simulink model "Digflt"  (Simulink 3.00)
settings: Solver=ode45  StartTime=0.0  StopTime=10.0  RelTol=1e-3
libraries: Dequiv x15, simulink3 x1
settings Model: LastModifiedBy=campa

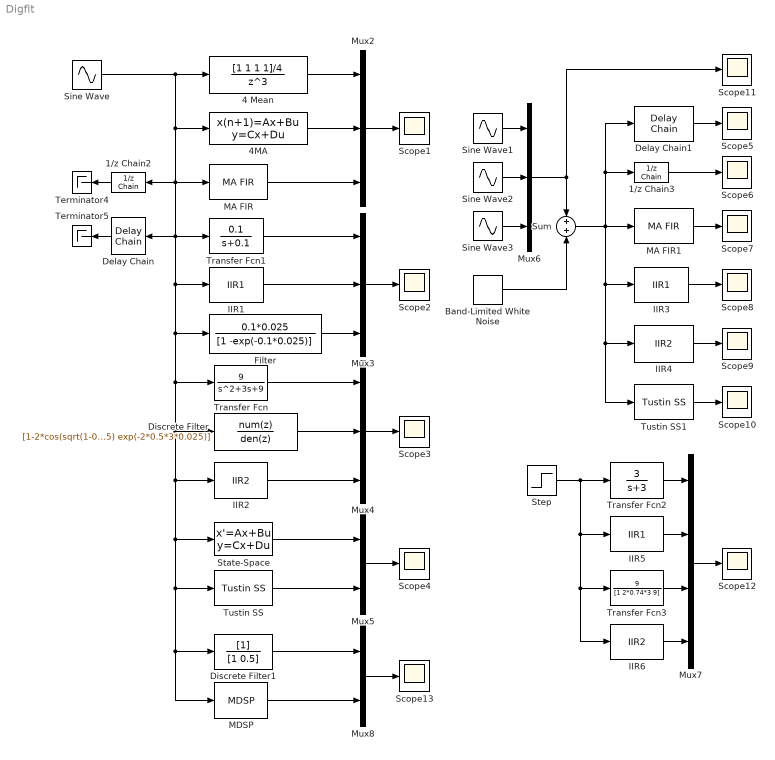
== system Digflt ==
  1/z Chain2 : Dequiv/1//z Chain  Orientation=left  ni=1  rd=4  x0=0  T=0.025
  1/z Chain3 : Dequiv/1//z Chain  ni=3  rd=4  x0=0  T=0.025
  4 Mean : DiscreteTransferFcn  Numerator=[1 1 1 1]/4  Denominator=[1 0 0 0]  SampleTime=0.025
  4MA : DiscreteStateSpace  A=[0 1 0;0 0 1;0 0 0]  B=[0 0 1/4]'  C=[1 1 1]  D=1/4  X0=0  SampleTime=0.025
  Band-Limited White Noise : simulink3/Sources/Band-Limited White Noise  Cov=0.01*ones(3,1)  Ts=0.025  seed=[1 2 3]
  Delay Chain : Dequiv/Delay Chain  Orientation=left  ni=1  rd=3  x0=2e-7/4  T=0.025
  Delay Chain1 : Dequiv/Delay Chain  ni=3  rd=3  x0=2e-7/4  T=0.025
  Discrete Filter : DiscreteFilter  Numerator=[1-2*cos(sqrt(1-0.5^2)*3*0.025)*exp(-0.5*3*0.025)+exp(-2*0.5*3*0.025)]  Denominator=[1 -2*cos(sqrt(1-0.5^2)*3*0.025)*exp(-0.5*3*0.025) exp(-2*0.5*3*0.025)]  SampleTime=0.025
  Discrete Filter1 : DiscreteFilter  Numerator=[1]  Denominator=[1 0.5]  SampleTime=0.025
  Filter : DiscreteFilter  Numerator=0.1*0.025  Denominator=[1 -exp(-0.1*0.025)]  SampleTime=0.025
  IIR1 : Dequiv/IIR1  ni=1  a=0.1  x0=0  T=0.025
  IIR2 : Dequiv/IIR2  ni=1  w=3  x=0.5  x0=0  T=0.025
  IIR3 : Dequiv/IIR1  ni=3  a=3  x0=0  T=0.025
  IIR4 : Dequiv/IIR2  ni=3  w=3  x=0.74  x0=0  T=0.025
  IIR5 : Dequiv/IIR1  ni=1  a=3  x0=0  T=0.025
  IIR6 : Dequiv/IIR2  ni=1  w=3  x=0.74  x0=0  T=0.025
  MA FIR : Dequiv/MA FIR  ni=1  ws=4  x0=2e-7/4  T=0.025
  MA FIR1 : Dequiv/MA FIR  ni=3  ws=4  x0=2e-7/4  T=0.025
  MDSP : Dequiv/MDSP  ni=1  num=[1 0]  den=[1 0.5]  u0=0  T=0.025
  Mux{2..4,6} (4 alike) : Mux  Inputs=3
  Mux5 : Mux  Inputs=2
  Mux7 : Mux  Inputs=4
  Mux8 : Mux  Inputs=2
  Scope{1..13} (13 alike) : Scope
      Scope1 settings: TimeRange=10  YMin=-1  YMax=1  SaveToWorkspace=off  SaveName=ScopeData
      Scope10 settings: TimeRange=10  YMin=-1  YMax=1  SaveToWorkspace=off  SaveName=ScopeData
      Scope11 settings: TimeRange=10  YMin=-1  YMax=1  SaveToWorkspace=off  SaveName=ScopeData
      Scope12 settings: TimeRange=10  YMin=0  YMax=1.5  SaveToWorkspace=off  SaveName=ScopeData
      Scope13 settings: TimeRange=10  YMin=-1  YMax=1  SaveToWorkspace=off  SaveName=ScopeData
      Scope2 settings: TimeRange=10  YMin=-0.05  YMax=0.15  SaveToWorkspace=off  SaveName=ScopeData
      Scope3 settings: TimeRange=10  YMin=-2  YMax=2  SaveToWorkspace=off  SaveName=ScopeData
      Scope4 settings: TimeRange=10  YMin=-1  YMax=1  SaveToWorkspace=off  SaveName=ScopeData
      Scope5 settings: TimeRange=10  YMin=-4  YMax=4  SaveToWorkspace=off  SaveName=ScopeData
      Scope6 settings: TimeRange=10  YMin=-4  YMax=4  SaveToWorkspace=off  SaveName=ScopeData
      Scope7 settings: TimeRange=10  YMin=-2  YMax=2  SaveToWorkspace=off  SaveName=ScopeData
      Scope8 settings: TimeRange=10  YMin=-1  YMax=1  SaveToWorkspace=off  SaveName=ScopeData
      Scope9 settings: TimeRange=10  YMin=-1  YMax=1  SaveToWorkspace=off  SaveName=ScopeData
  Sine Wave : Sin  Amplitude=1  Frequency=2  Phase=0  SampleTime=0
  Sine Wave1 : Sin  Amplitude=1  Frequency=1.5  Phase=0  SampleTime=0
  Sine Wave2 : Sin  Amplitude=1  Frequency=1.5  Phase=pi/4  SampleTime=0
  Sine Wave3 : Sin  Amplitude=1  Frequency=1.5  Phase=pi/2  SampleTime=0
  State-Space : StateSpace  A=[0 1;-3^2 -2*3*0.74]  B=[0;3^2]  C=[1 0]  D=0  X0=0
  Step : Step  Time=1  Before=0  After=1  SampleTime=0
  Sum : Sum  Inputs=++  SaturateOnIntegerOverflow=on
  Terminator4 : Terminator
  Terminator5 : Terminator
  Transfer Fcn : TransferFcn  Numerator=9  Denominator=[1 3 9]
  Transfer Fcn1 : TransferFcn  Numerator=0.1  Denominator=[1 0.1]
  Transfer Fcn2 : TransferFcn  Numerator=3  Denominator=[1 3]
  Transfer Fcn3 : TransferFcn  Numerator=9  Denominator=[1 2*0.74*3 9]
  Tustin SS : Dequiv/Tustin SS  n=1  a=[0 1;-3^2 -2*3*0.74]  b=[0;3^2]  c=[1 0]  d=0  w=1  u0=0  T=0.025
  Tustin SS1 : Dequiv/Tustin SS  n=3  a=[0 1;-3^2 -2*3*0.74]  b=[0;3^2]  c=[1 0]  d=0  w=1  u0=0  T=0.025
  wires:
  Mux2/1 -> Scope1/1
  MA FIR/1 -> Mux2/3
  Sine Wave/1 -> 4 Mean/1, 4MA/1, MA FIR/1, Transfer Fcn1/1, IIR1/1, Transfer Fcn/1, Discrete Filter/1, IIR2/1, State-Space/1, Tustin SS/1, Discrete Filter1/1, MDSP/1, Filter/1, Delay Chain/1, 1/z Chain2/1
  4 Mean/1 -> Mux2/1
  4MA/1 -> Mux2/2
  1/z Chain2/1 -> Terminator4/1
  1/z Chain3/1 -> Scope6/1
  Delay Chain1/1 -> Scope5/1
  IIR3/1 -> Scope8/1
  Tustin SS1/1 -> Scope10/1
  MA FIR1/1 -> Scope7/1
  IIR4/1 -> Scope9/1
  Sum/1 -> MA FIR1/1, IIR3/1, IIR4/1, Tustin SS1/1, 1/z Chain3/1, Delay Chain1/1
  Band-Limited White Noise/1 -> Sum/2
  Sine Wave1/1 -> Mux6/1
  Sine Wave2/1 -> Mux6/2
  Sine Wave3/1 -> Mux6/3
  Mux6/1 -> Sum/1, Scope11/1
  Transfer Fcn2/1 -> Mux7/1
  IIR5/1 -> Mux7/2
  Transfer Fcn3/1 -> Mux7/3
  IIR6/1 -> Mux7/4
  Step/1 -> Transfer Fcn2/1, IIR5/1, Transfer Fcn3/1, IIR6/1
  Mux7/1 -> Scope12/1
  Mux3/1 -> Scope2/1
  Transfer Fcn1/1 -> Mux3/1
  IIR1/1 -> Mux3/2
  Filter/1 -> Mux3/3
  Delay Chain/1 -> Terminator5/1
  IIR2/1 -> Mux4/3
  Mux4/1 -> Scope3/1
  Discrete Filter/1 -> Mux4/2
  Transfer Fcn/1 -> Mux4/1
  Mux5/1 -> Scope4/1
  State-Space/1 -> Mux5/1
  Tustin SS/1 -> Mux5/2
  Discrete Filter1/1 -> Mux8/1
  MDSP/1 -> Mux8/2
  Mux8/1 -> Scope13/1
